simulink model "lanedetection_rgb"  (R2018a)
settings: Solver=FixedStepAuto  StartTime=0.0  StopTime=inf  RelTol=1e-3  EnableMultiTasking=on
undefined symbols (not defined in the file): gray, Rec, SDTV
libraries: visiontransforms x2, embdlinuxlib x2, dspmtrx3 x2, visionconversions x1, visiontextngfix x1, visionanalysis x1, visionstatistics x1
settings Model: SimulationMode=external  Creator=ifadmin  LastModifiedBy=ifadmin
settings SolverCC: PositivePriorityOrder=on
settings OptimizationCC: EnhancedBackFolding=on  PassReuseOutputArgsAs=Individual arguments  MaxStackSize=64  OptimizeBlockOrder=speed  DifferentSizesBufferReuse=on  OptimizationCustomize=off
settings DebuggingCC: ParameterOverflowMsg=warning  ParameterTunabilityLossMsg=error
settings HardwareCC: ProdBitPerPointer=32  ProdBitPerSizeT=32  ProdBitPerPtrDiffT=32  ProdLargestAtomicInteger=Long  ProdLargestAtomicFloat=Double  ProdWordSize=32  ProdHWDeviceType=ARM Compatible->ARM Cortex
settings SFSimCC: MATLABDynamicMemAlloc=off
settings RTWCC: SystemTargetFile=ert.tlc  HardwareBoard=Raspberry Pi  TLCOptions="-aInlineSetEventsForThisBaseRateFcn=TLC_FALSE -aSuppressMultiTaskScheduler=TLC_FALSE  -aRateBasedStepFcn=0"  TemplateMakefile=ert_default_tmf  GenerateReport=on  Toolchain=GNU GCC Raspberry Pi  BuildConfiguration=Faster Runs  IncludeHyperlinkInReport=on  LaunchReport=on  GenerateTraceInfo=on  GenerateTraceReport=on  GenerateTraceReportSl=on  GenerateTraceReportSf=on  GenerateTraceReportEml=on
settings CodeAppCC: ForceParamTrailComments=on  IgnoreCustomStorageClasses=off  OperatorAnnotations=on  SimulinkDataObjDesc=on  SFDataObjDesc=on  InsertBlockDesc=on
settings ERTTargetCC: SupportVariableSizeSignals=on

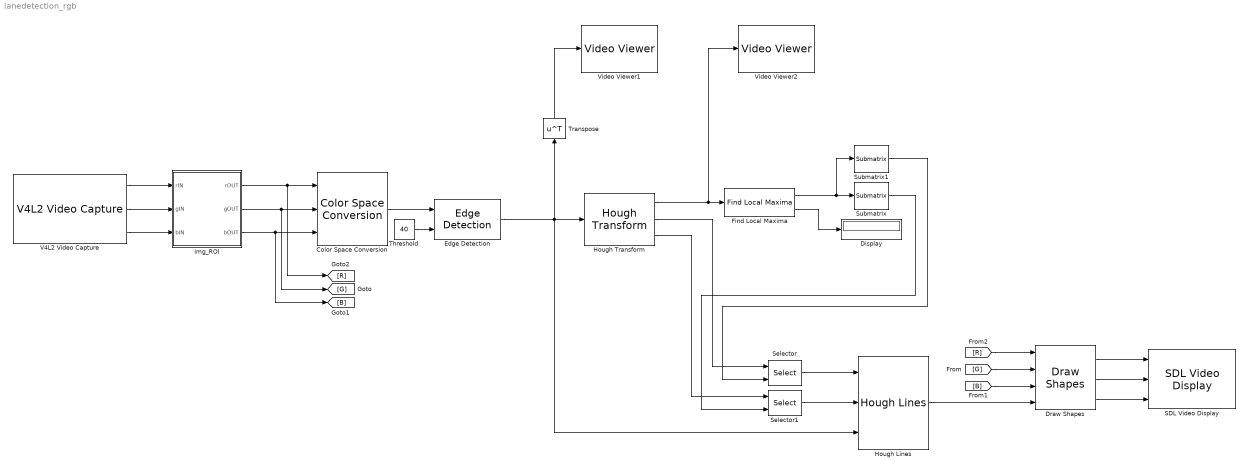
== system lanedetection_rgb ==
  Color Space Conversion : visionconversions/Color Space  Conversion  conversion=Obsolete  conversionActive=R'G'B' to intensity  wp_str=D65  rec=Rec. 601 (SDTV)  sys=1125/60/2:1  imagePorts=Separate color signals
      settings: SourceProductName=Computer Vision System Toolbox
  Display : Display
  Draw Shapes : visiontextngfix/Draw Shapes  shape=Lines  fill=off  lineWidth=2  fillClrSource=Specify via dialog  display=User-specified value  intensity=200  color=[255 000 000]  opacity=0.6  viewport=Entire image  antialiasing=off  inType=Obsolete  imagePorts=Separate color signals  prodOutputMode=Binary point scaling  prodOutputWordLength=32  prodOutputFracLength=14  memoryMode=Specify word length  memoryWordLength=16  memoryFracLength=14  roundingMode=Floor  overflowMode=off
      settings: SourceProductName=Computer Vision System Toolbox  LockScale=on
  Edge Detection : visionanalysis/Edge Detection  method=Sobel  outputType=Binary image  userDefinedThreshold=on  thresholdSource=Input port  threshold=20  thresholdTuning=4  edgeThinning=on  threshold_canny=[0.25 0.60]  autoPercent=70  sigma=1  roundingMode=Floor  overflowMode=off  prodOutputMode=Binary point scaling  prodOutputWordLength=32  prodOutputFracLength=8  prodOutputSlope=2^-8  accumSlope=2^-8  outputSlope=2^-4
      settings: SourceProductName=Computer Vision System Toolbox  SourceProductBaseCode=VP
  Find Local Maxima : visionstatistics/Find Local Maxima  num_peaks=2  nhood_size=[45 25]  src_thresh=Obsolete9b  src_thresh_inuse=Specify via dialog  threshold=20  inputIsHough=on  dt_peak=single  isOutVarDim=off  dt_count=single
      settings: SourceProductName=Computer Vision System Toolbox  SourceProductBaseCode=VP
  Hough Lines : visiontransforms/Hough Lines  sineCompMethod=Trigonometric function  thetaRes=pi/180  firstCoeffMode=Specify word length  firstCoeffWordLength=16  firstCoeffFracLength=15  prodOutputMode=Binary point scaling  prodOutputWordLength=32  prodOutputFracLength=16  roundingMode=Nearest  overflowMode=on
      settings: SourceProductName=Computer Vision System Toolbox  SourceProductBaseCode=VP
  Hough Transform : visiontransforms/Hough Transform  theta_res=pi/90  rho_res=4  out_theta_rho=on  outdtmode=single  firstCoeffMode=Binary point scaling  firstCoeffWordLength=16  firstCoeffFracLength=14  secondCoeffMode=Binary point scaling  secondCoeffWordLength=32  secondCoeffFracLength=16  outputMode=Binary point scaling  outputWordLength=16  outputFracLength=0  accumMode=Binary point scaling  accumWordLength=32  accumFracLength=20  prodOutputMode=Binary point scaling  prodOutputWordLength=32  prodOutputFracLength=20  memoryMode=Binary point scaling  memoryWordLength=32  memoryFracLength=16  roundingMode=Nearest  overflowMode=on
      settings: SourceProductName=Computer Vision System Toolbox  SourceProductBaseCode=VP
  SDL Video Display : embdlinuxlib/SDL Video Display  pixelFormat=RGB  pixelOrder=Planar  rowMajor=on  blockPlatform=Raspberry Pi
      settings: SourceProductName=Simulink Support Package for Raspberry Pi Hardware  SourceProductBaseCode=RASPPI
  Selector : Selector  InputPortWidth=90  IndexOptions=Index vector (port)  Indices=[1 3]  OutputSizes=46
  Selector1 : Selector  InputPortWidth=163  IndexOptions=Index vector (port)  Indices=[1 3]  OutputSizes=1
  Submatrix : dspmtrx3/Submatrix  RowSpan=All rows  RowStartMode=Last  RowStartIndex=1  RowEndMode=Last  RowEndIndex=1  ColSpan=One column  ColStartMode=Last  ColStartIndex=1  ColEndMode=Last  ColEndIndex=1
  Submatrix1 : dspmtrx3/Submatrix  RowSpan=All rows  RowStartMode=First  RowStartIndex=1  RowEndMode=Offset from last  RowEndIndex=1  ColSpan=One column  ColStartMode=First  ColStartIndex=1  ColEndMode=Last  ColEndIndex=1
  Threshold : Constant  Value=40  OutDataTypeStr=uint8  LockScale=on
  Transpose : Math  Operator=transpose  SaturateOnIntegerOverflow=on
  V4L2 Video Capture : embdlinuxlib/V4L2 Video Capture  m_devName='/dev/video0'  roi=[0, 0, 640, 480]  imSizeSelection=320x240  imSize=[640, 480]  pixelFormat=RGB  pixelOrder=Planar  sampleTime=1/10  simOutput=Colorbars  blockPlatform=Raspberry Pi
      settings: SourceProductName=Simulink Support Package for Raspberry Pi Hardware  SourceProductBaseCode=RASPPI
  Video Viewer1 : VideoViewer  colormapValue=gray(256)  FigPos=[1922 882 958 469]
  Video Viewer2 : VideoViewer  colormapValue=gray(256)  FigPos=[2882 882 958 1049]
  img_ROI : MATLAB Function  TreatAsAtomicUnit=on
  wires:
  Hough Transform/2 -> Selector/1
  Hough Transform/3 -> Selector1/1
  Selector/1 -> Hough Lines/1
  Submatrix1/1 -> Selector/2
  Find Local Maxima/2 -> Display/1
  Submatrix/1 -> Selector1/2
  Threshold/1 -> Edge Detection/2
  Color Space Conversion/1 -> Edge Detection/1
  img_ROI/1(rOUT) -> Color Space Conversion/1, [R]
  img_ROI/2(gOUT) -> Color Space Conversion/2, [G]
  img_ROI/3(bOUT) -> Color Space Conversion/3, [B]
  Edge Detection/1 -> Transpose/1, Hough Transform/1, Hough Lines/3
  Transpose/1 -> Video Viewer1/1
  V4L2 Video Capture/1 -> img_ROI/1(rIN)
  V4L2 Video Capture/2 -> img_ROI/2(gIN)
  V4L2 Video Capture/3 -> img_ROI/3(bIN)
  Draw Shapes/1 -> SDL Video Display/1
  Draw Shapes/2 -> SDL Video Display/2
  Draw Shapes/3 -> SDL Video Display/3
  Hough Lines/1 -> Draw Shapes/4
  Selector1/1 -> Hough Lines/2
  [R] -> Draw Shapes/1
  [G] -> Draw Shapes/2
  [B] -> Draw Shapes/3
  Hough Transform/1 -> Video Viewer2/1, Find Local Maxima/1
  Find Local Maxima/1 -> Submatrix1/1, Submatrix/1

== matlab function lanedetection_rgb/img_ROI ==
  data: rIN input uint8 size=[320 240]; rOUT output uint8 size=[316 70]; gIN input size=[320 240]; bIN input size=[320 240]; gOUT output size=[316 70]; bOUT output size=[316 70]
function [rOUT, gOUT, bOUT]  = imgROI(rIN, gIN, bIN)

    % 160x120
    %rOUT = rIN(2:159, 48:83);
    %gOUT = gIN(2:159, 48:83);
    %bOUT = bIN(2:159, 48:83);
    
    % 320 x 240
    rOUT = rIN(3:318, 96:165);
    gOUT = gIN(3:318, 96:165);
    bOUT = bIN(3:318, 96:165);
    
    % 800 x 600
    %imgOUT = imgIN(0:799 ,300:499);

end
